simulink subsystem "sensors"  (R2026a)
settings: Solver=VariableStepAuto
undefined symbols (not defined in the file): imu1_accel_bias, imu1_accel_noise, imu1_gyro_bias, imu1_gyro_noise, imu1_mag_noise, imu2_accel_bias, imu2_accel_noise, imu2_gyro_bias, imu2_gyro_noise, imu2_mag_noise, imu3_accel_bias, imu3_accel_noise, imu3_gyro_bias, imu3_gyro_noise
settings Model: Creator=joedo  LastModifiedBy=trist

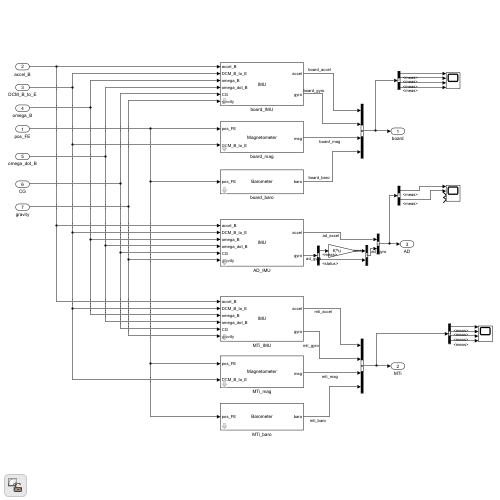
[thumbnail: Simulink's stored preview of the top-level diagram]
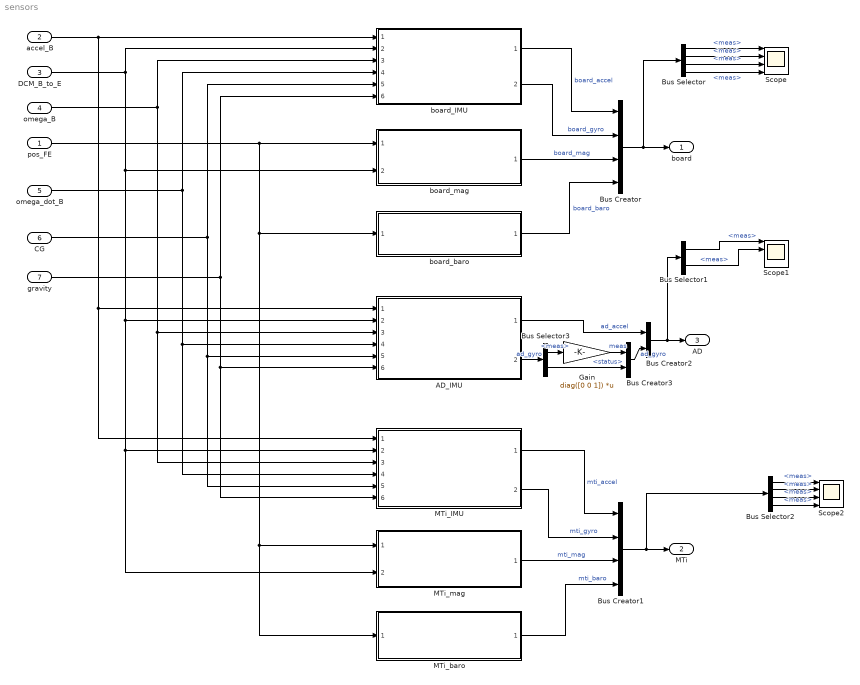
== system sensors ==
  pos_FE : Inport
  accel_B : Inport  Port=2
  DCM_B_to_E : Inport  Port=3
  omega_B : Inport  Port=4
  omega_dot_B : Inport  Port=5
  CG : Inport  Port=6
  gravity : Inport  Port=7
  AD_IMU : Subsystem  ReferencedSubsystem=sensor_imu  samplingrate=samplingtime_imu  noise_accel=imu3_accel_noise * [1,1,1]  bias_accel=imu3_accel_bias * [1 1 1]  scale_accel=[1 0 0; 0 1 0; 0 0 1]  lim_accel=imu3_accel_limit  noise_gyro=imu3_gyro_noise * [1 1 1]  bias_gyro=imu3_gyro_bias * [1 1 1]  scale_gyro=[1 0 0; 0 1 0; 0 0 1]  lim_gyro=imu3_gyro_limit  S=sensor_3_S  d=sensor_3_d
  Bus Creator : BusCreator  Inputs=4
  Bus Creator1 : BusCreator  Inputs=4
  Bus Creator2 : BusCreator  Inputs=2
  Bus Creator3 : BusCreator  Inputs=2
  Bus Selector : BusSelector  OutputSignals=board_accel.meas,board_gyro.meas,board_mag.meas,board_baro.meas
  Bus Selector1 : BusSelector  OutputSignals=ad_accel.meas,ad_gyro.meas
  Bus Selector2 : BusSelector  OutputSignals=mti_accel.meas,mti_gyro.meas,mti_mag.meas,mti_baro.meas
  Bus Selector3 : BusSelector  OutputSignals=meas,status
  Gain : Gain  Gain=diag([0 0 1])  Multiplication=Matrix(K*u)
  MTi_IMU : Subsystem  ReferencedSubsystem=sensor_imu  samplingrate=samplingtime_imu  noise_accel=imu2_accel_noise * [1 1 1]  bias_accel=imu2_accel_bias * [1 1 1]  scale_accel=[1 0 0; 0 1 0; 0 0 1]  lim_accel=imu2_accel_limit  noise_gyro=imu2_gyro_noise * [1 1 1]  bias_gyro=imu2_gyro_bias * [1 1 1]  scale_gyro=[1 0 0; 0 1 0; 0 0 1]  lim_gyro=imu2_gyro_limit  S=sensor_2_S  d=sensor_2_d
  MTi_baro : Subsystem  ReferencedSubsystem=sensor_baro  samplingrate=samplingtime_other  noise_pres=imu2_baro_noise  bias_pres=imu2_baro_bias  scale_pres=1  limit_pres=imu2_baro_limit
  MTi_mag : Subsystem  ReferencedSubsystem=sensor_mag  samplingrate=samplingtime_other  noise_mag=imu2_mag_noise * [1 1 1]  bias_mag=[0 0 0]  scale_mag=[1 0 0; 0 1 0; 0 0 1]  limit_mag=imu2_mag_limit  Ssi=sensor_2_S  Lsi=sensor_1_d  lon=80.5204  lat=43.4643  year=2025
  Scope : Scope  NumInputPorts=4
      settings: ActiveDisplayYMinimum=-11.169561599813589  ActiveDisplayYMaximum=2.5675021643770561  DataLoggingVariableName=ScopeData12
  Scope1 : Scope  NumInputPorts=4
      settings: ActiveDisplayYMinimum=-57.597626786179724  ActiveDisplayYMaximum=116.9562021436104  DataLoggingVariableName=ScopeData13
  Scope2 : Scope  NumInputPorts=4
      settings: ActiveDisplayYMinimum=-72.9345654611225  ActiveDisplayYMaximum=117.10384060679139  DataLoggingVariableName=ScopeData18
  board_IMU : Subsystem  ReferencedSubsystem=sensor_imu  samplingrate=samplingtime_imu  noise_accel=imu1_accel_noise * [1,1,1]  bias_accel=imu1_accel_bias * [1 1 1]  scale_accel=[1 0 0; 0 1 0; 0 0 1]  lim_accel=imu1_accel_limit  noise_gyro=imu1_gyro_noise * [1,1,1]  bias_gyro=imu1_gyro_bias * [1 1 1]  scale_gyro=[1 0 0; 0 1 0; 0 0 1]  lim_gyro=imu1_gyro_limit  S=sensor_1_S_acc  d=sensor_1_d
  board_baro : Subsystem  ReferencedSubsystem=sensor_baro  samplingrate=samplingtime_other  noise_pres=imu1_baro_noise  bias_pres=imu1_baro_bias  scale_pres=1  limit_pres=imu1_baro_limit
  board_mag : Subsystem  ReferencedSubsystem=sensor_mag  samplingrate=samplingtime_other  noise_mag=imu1_mag_noise * [1,1,1]  bias_mag=[0 0 0]  scale_mag=[1 0 0; 0 1 0; 0 0 1]  limit_mag=imu1_mag_limit  Ssi=sensor_1_S_mag  Lsi=sensor_1_d  lon=80.5204  lat=43.4643  year=2025
  board : Outport
  MTi : Outport  Port=2
  AD : Outport  Port=3
  wires:
  Bus Creator/1 -> board/1, Bus Selector/1
  board_baro/1 -> Bus Creator/4  "board_baro"
  MTi_baro/1 -> Bus Creator1/4  "mti_baro"
  MTi_IMU/1 -> Bus Creator1/1  "mti_accel"
  MTi_mag/1 -> Bus Creator1/3  "mti_mag"
  AD_IMU/1 -> Bus Creator2/1  "ad_accel"
  accel_B/1 -> MTi_IMU/1, AD_IMU/1, board_IMU/1
  omega_B/1 -> MTi_IMU/3, AD_IMU/3, board_IMU/3
  omega_dot_B/1 -> MTi_IMU/4, AD_IMU/4, board_IMU/4
  CG/1 -> MTi_IMU/5, AD_IMU/5, board_IMU/5
  gravity/1 -> MTi_IMU/6, AD_IMU/6, board_IMU/6
  MTi_IMU/2 -> Bus Creator1/2  "mti_gyro"
  board_IMU/1 -> Bus Creator/1  "board_accel"
  board_IMU/2 -> Bus Creator/2  "board_gyro"
  Bus Selector/1 -> Scope/1  "<meas>"
  Bus Selector/2 -> Scope/2  "<meas>"
  Bus Selector/3 -> Scope/3  "<meas>"
  Bus Selector/4 -> Scope/4  "<meas>"
  Bus Selector1/1 -> Scope1/1  "<meas>"
  Bus Creator2/1 -> AD/1, Bus Selector1/1
  Bus Selector1/2 -> Scope1/2  "<meas>"
  Bus Selector2/4 -> Scope2/4  "<meas>"
  Bus Selector2/3 -> Scope2/3  "<meas>"
  Bus Selector2/2 -> Scope2/2  "<meas>"
  Bus Creator1/1 -> MTi/1, Bus Selector2/1
  Bus Selector2/1 -> Scope2/1  "<meas>"
  DCM_B_to_E/1 -> board_IMU/2, MTi_mag/2, MTi_IMU/2, AD_IMU/2, board_mag/2
  pos_FE/1 -> MTi_baro/1, MTi_mag/1, board_baro/1, board_mag/1
  board_mag/1 -> Bus Creator/3  "board_mag"
  AD_IMU/2 -> Bus Selector3/1  "ad_gyro"
  Gain/1 -> Bus Creator3/1  "meas"
  Bus Selector3/1 -> Gain/1  "<meas>"
  Bus Selector3/2 -> Bus Creator3/2  "<status>"
  Bus Creator3/1 -> Bus Creator2/2  "ad_gyro"
